simulink model "udptestR2021a"  (R2021a)
settings: Solver=FixedStepAuto  StartTime=0.0  StopTime=10.0  FixedStep=1  RelTol=1e-3
libraries: dspnetwork x2
settings Model: EnablePacing=on  Creator=Claire  LastModifiedBy=Administrator
settings DebuggingCC: UnconnectedInputMsg=none  UnconnectedOutputMsg=none  UnconnectedLineMsg=none
settings ModelReferenceCC: EnableRefExpFcnMdlSchedulingChecks=off
settings RTWCC: Description=Generic Real-Time Target  DLArmComputeVersion=20.02.1

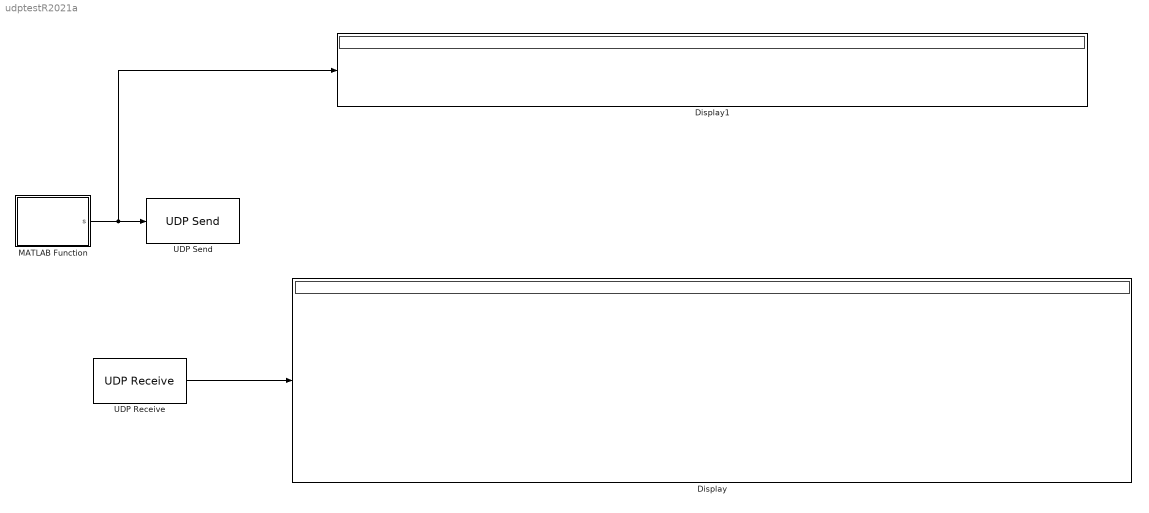
== system udptestR2021a ==
  Display : Display
  Display1 : Display
  MATLAB Function : MATLAB Function  TreatAsAtomicUnit=on
  UDP Receive : dspnetwork/UDP Receive  localURL='0.0.0.0'  localPort=9798  remoteURL='0.0.0.0'  remotePort=-1  recvBufferSize=8192  dims=255  signalDatatype=double  isComplex=off  isVarSize=on  showBlockingTime=off  blockingTime=0  sampletime=1  blockPlatform=[]
  UDP Send : dspnetwork/UDP Send  remoteURL='127.0.0.1'  remotePort=9797  localURL='0.0.0.0'  localPortSource=Automatically determine  localPort=-1  sendBufferSize=8192  sampletime=-1  blockPlatform=[]  separateLengthPort=0
  wires:
  MATLAB Function/1(s) -> UDP Send/1, Display1/1
  UDP Receive/1 -> Display/1

== matlab function udptestR2021a/MATLAB Function ==
  data: s output
function s = fcn()
%发送格式【Pcur（100x3）；p_search（50x3）】
Pcur=[
69450.0210628131	73209.7717279049	3000;
69109.1259625001	73166.1601007052	3000;
68725.7794490756	72915.1248806007	3000;
68276.9772450387	72722.5747908658	3000;
69336.0168977699	72840.5185836608	3000;
68970.0024341455	72650.1482374550	3000;
68493.4979439884	72441.3907880869	3000;
68120.5158221452	72270.6558342081	3000;
69113.8330730040	72346.0460930507	3000;
68740.3847813767	72189.1429330583	3000;
68309.2838154941	71962.5195493329	3000;
67983.4409519468	71853.9705747478	3000;
69035.0211759836	72014.9133955126	3000;
68632.0837389493	71858.0139388334	3000;
25772.3673509756	76274.0311161872	3000;
25839.0995139336	75943.4452376875	3000;
27311.7813214795	74929.7969880627	3000;
27089.3700808911	74637.4981299963	3000;
27120.5966446095	76037.7348916201	3000;
27456.5666822007	75866.5832970368	3000;
31427.5314364911	77035.9521198638	3000;
31331.6486294013	76722.6841435341	3000;
29796.1252660496	77935.6580698348	3000;
29554.4378179295	77499.7398861929	3000;
30399.4544789689	76714.7301718913	3000;
30466.4614534937	76402.3534641907	3000;
30062.6706052765	77512.3390274549	3000;
50576.8333764787	16916.2320273949	3000;
52306.5357451163	15929.2740466941	3000;
52156.4138267135	15646.5880060671	3000;
53005.5688689737	15341.9616096527	3000;
51859.1869625078	16797.7662273930	3000;
53643.5069682220	16010.8839710945	3000;
53447.3905956578	15760.2430659532	3000;
53214.5850731798	15564.4591821436	3000;
52013.6417244321	17078.4102415038	3000;
53705.4229870906	15739.4592871936	3000;
53385.1912993352	16278.8114574284	3000;
53751.9910870910	16295.3807416653	3000;
52307.3790057990	17158.3975324823	3000;
zeros(60,3)];
p_search = [
 68631.0254764935	71934.1965695342 3000;
 23289.8902697303	77582.9094928906 3000;
 61360.6274638467	11770.4961848512 3000;
 69642.1290954389	37021.1199980277 3000;
 11970.2298166359	31692.6592293240 3000;
 50332.1647144018	54810.8833394563 3000;
 zeros(44,3)];
s=[Pcur',p_search'];
